simulink model "AeroCoeffsNew"  (R2020b)
settings: Solver=VariableStepAuto  StartTime=0.0  StopTime=50  FixedStep=0.1  RelTol=1e-3
values from neighbouring files (symbols this model uses):
  A_2 = [0  0  0; 0  0  0; 0  0  0]    [Angular_gust.mat]    (also in Linear_gust.mat; Real_Values.m = zeros(3); Trial_Script.m = zeros(3); TryingNewAeroCoeffs.m = zeros(3))
  A_kal = [0 0 0 0 0 0 0 0 0 0 0 0 ... (36 elements, 6x6)]    [Angular_gust.mat]    (also in Linear_gust.mat; Real_Values.m = [0 0 0 1 0 0; Trial_Script.m = [0 0 0 1 0 0; TryingNewAeroCoeffs.m = [0 0 0 1 0 0)
  B_2 = [0.0024294842205  2.57653534931e-06  6.44659625064e-05; 0  -0.000916808772026  -2.10833406567e-07; 0  0  -0.000799328564006]    [Angular_gust.mat]    (also in Linear_gust.mat; Real_Values.m = I_inv; Trial_Script.m = I_inv; TryingNewAeroCoeffs.m = I_inv)
  B_kal = [0 0 0 0 0 0 0 0 0 0 0 0 ... (36 elements, 6x6)]    [Angular_gust.mat]    (also in Linear_gust.mat; Real_Values.m = [0 0 0 0 0 0; Trial_Script.m = [0 0 0 0 0 0; TryingNewAeroCoeffs.m = [0 0 0 0 0 0)
  C_2 = [1  0  0; 0  1  0; 0  0  1]    [Angular_gust.mat]    (also in Linear_gust.mat; Real_Values.m = eye(3); Trial_Script.m = eye(3); TryingNewAeroCoeffs.m = eye(3))
  C_kal = [1 0 0 0 0 0 0 1 0 0 0 0 ... (36 elements, 6x6)]    [Angular_gust.mat]    (also in Linear_gust.mat; Real_Values.m = eye(6); Trial_Script.m = eye(6); TryingNewAeroCoeffs.m = eye(6))
  D_2 = [0  0  0; 0  0  0; 0  0  0]    [Angular_gust.mat]    (also in Linear_gust.mat; Real_Values.m = zeros(3); Trial_Script.m = zeros(3); TryingNewAeroCoeffs.m = zeros(3))
  D_kal = [0 0 0 0 0 0 0 0 0 0 0 0 ... (36 elements, 6x6)]    [Angular_gust.mat]    (also in Linear_gust.mat; Real_Values.m = zeros(6); Trial_Script.m = zeros(6); TryingNewAeroCoeffs.m = zeros(6))
  delta_time = 0.0178961433409    [Angular_gust.mat]    (also in Linear_gust.mat; Real_Values.m = time/length(xdata); Trial_Script.m = time/length(xdata); TryingNewAeroCoeffs.m = time/length(xdata))
  Fb1_l = -2600    [Angular_gust.mat]    (also in Linear_gust.mat; Real_Values.m = -260; Trial_Script.m; TryingNewAeroCoeffs.m)
  Fb1_u = 2600    [Angular_gust.mat]    (also in Linear_gust.mat; Real_Values.m = 260; Trial_Script.m; TryingNewAeroCoeffs.m)
  Fb2_l = -2600    [Angular_gust.mat]    (also in Linear_gust.mat; Real_Values.m = -260; Trial_Script.m; TryingNewAeroCoeffs.m)
  Fb2_u = 2600    [Angular_gust.mat]    (also in Linear_gust.mat; Real_Values.m = 260; Trial_Script.m; TryingNewAeroCoeffs.m)
  Fb3_l = -3200    [Angular_gust.mat]    (also in Linear_gust.mat; Real_Values.m = -320; Trial_Script.m; TryingNewAeroCoeffs.m)
  Fb3_u = 3200    [Angular_gust.mat]    (also in Linear_gust.mat; Real_Values.m = 320; Trial_Script.m; TryingNewAeroCoeffs.m)
  Fb4_l = -3200    [Angular_gust.mat]    (also in Linear_gust.mat; Real_Values.m = -320; Trial_Script.m; TryingNewAeroCoeffs.m)
  Fb4_u = 3200    [Angular_gust.mat]    (also in Linear_gust.mat; Real_Values.m = 320; Trial_Script.m; TryingNewAeroCoeffs.m)
  Fc1_l = -300    [Angular_gust.mat]    (also in Linear_gust.mat; Real_Values.m = -100; Trial_Script.m = -3000; TryingNewAeroCoeffs.m)
  Fc1_u = 300    [Angular_gust.mat]    (also in Linear_gust.mat; Real_Values.m = 100; Trial_Script.m = 3000; TryingNewAeroCoeffs.m)
  Fc2_l = -300    [Angular_gust.mat]    (also in Linear_gust.mat; Real_Values.m = -100; Trial_Script.m = -3000; TryingNewAeroCoeffs.m)
  Fc2_u = 300    [Angular_gust.mat]    (also in Linear_gust.mat; Real_Values.m = 100; Trial_Script.m = 3000; TryingNewAeroCoeffs.m)
  Fc3_l = -300    [Angular_gust.mat]    (also in Linear_gust.mat; Real_Values.m = -100; Trial_Script.m = -3000; TryingNewAeroCoeffs.m)
  Fc3_u = 300    [Angular_gust.mat]    (also in Linear_gust.mat; Real_Values.m = 100; Trial_Script.m = 3000; TryingNewAeroCoeffs.m)
  fprop = 1000    [Angular_gust.mat]    (also in Linear_gust.mat; TryingNewAeroCoeffs.m)
  Ft1_l = -5600    [Angular_gust.mat]    (also in Linear_gust.mat; Real_Values.m = -560; Trial_Script.m; TryingNewAeroCoeffs.m)
  Ft1_u = 5600    [Angular_gust.mat]    (also in Linear_gust.mat; Real_Values.m = 560; Trial_Script.m; TryingNewAeroCoeffs.m)
  Ft2_l = -5600    [Angular_gust.mat]    (also in Linear_gust.mat; Real_Values.m = -560; Trial_Script.m; TryingNewAeroCoeffs.m)
  Ft2_u = 5600    [Angular_gust.mat]    (also in Linear_gust.mat; Real_Values.m = 560; Trial_Script.m; TryingNewAeroCoeffs.m)
  Ft3_l = -3200    [Angular_gust.mat]    (also in Linear_gust.mat; Real_Values.m = -320; Trial_Script.m; TryingNewAeroCoeffs.m)
  Ft3_u = 3200    [Angular_gust.mat]    (also in Linear_gust.mat; Real_Values.m = 320; Trial_Script.m; TryingNewAeroCoeffs.m)
  Ft4_l = -3200    [Angular_gust.mat]    (also in Linear_gust.mat; Real_Values.m = -320; Trial_Script.m; TryingNewAeroCoeffs.m)
  Ft4_u = 3200    [Angular_gust.mat]    (also in Linear_gust.mat; Real_Values.m = 320; Trial_Script.m; TryingNewAeroCoeffs.m)
  g = 9.81    [Angular_gust.mat]    (also in Linear_gust.mat; Real_Values.m; Trial_Script.m; TryingNewAeroCoeffs.m)
  m = 941.102    [Angular_gust.mat]    (also in Linear_gust.mat; Real_Values.m; Trial_Script.m = 645; TryingNewAeroCoeffs.m)
  r_0 = [0 0 0]    [Angular_gust.mat]    (also in Linear_gust.mat; Real_Values.m = [0;0;0]; Trial_Script.m = [0;0;0]; TryingNewAeroCoeffs.m = [0;0;0])
  r_cgCatia = [0.0401998 0.00180957 -0.293434]    [Angular_gust.mat]    (also in Linear_gust.mat; Real_Values.m = TcgCatia*r_cgCatia; Trial_Script.m = [2; 0; 0]; TryingNewAeroCoeffs.m = TcgCatia*r_cgCatia)
  r_trajectory = [0 0 0]    [Angular_gust.mat]    (also in Linear_gust.mat; Real_Values.m = [0;0;0]; Trial_Script.m = [0;0;0]; TryingNewAeroCoeffs.m = [0;0;0])
  rho = 1.225    [Angular_gust.mat]    (also in Linear_gust.mat; Real_Values.m; Trial_Script.m; TryingNewAeroCoeffs.m)
  T = 10.5    [Angular_gust.mat]    (also in Linear_gust.mat; Real_Values.m; Trial_Script.m; TryingNewAeroCoeffs.m)
  t_finalgust = 17.9140394843    [Angular_gust.mat]    (also in Linear_gust.mat; Real_Values.m = time; TryingNewAeroCoeffs.m = time)
  TcgCatia = [1  0  0; 0  -1  0; 0  0  -1]    [Angular_gust.mat]    (also in Linear_gust.mat; Real_Values.m = [1 0 0; Trial_Script.m = [1 0 0; TryingNewAeroCoeffs.m = [1 0 0)
  time = 17.9140394843    [Angular_gust.mat]    (also in Linear_gust.mat; Real_Values.m = rdiff_abs/V0_shard; Trial_Script.m = abs(rdiff_shard(2)/V0_shard(2)); TryingNewAeroCoeffs.m = rdiff_abs/V0_shard)
  time_delay = 0.01    [Angular_gust.mat]    (also in Linear_gust.mat; Real_Values.m = 0.1; Trial_Script.m = 0.1; TryingNewAeroCoeffs.m)
  Tzy_Shard = [6.12323399574e-17  1  1.22464679915e-16; 1  -6.12323399574e-17  -7.49879891331e-33; 0  1.22464679915e-16  -1]    [Angular_gust.mat]    (also in Linear_gust.mat; Real_Values.m = [cos(pi/2) -sin(pi/2) 0; sin(pi/2) cos(pi/2) 0; 0 0 1]*[1 0 ; Trial_Script.m = [cos(pi/2) -sin(pi/2) 0; sin(pi/2) cos(pi/2) 0; 0 0 1]*[1 0 ; TryingNewAeroCoeffs.m = [cos(pi/2) -sin(pi/2) 0; sin(pi/2) cos(pi/2) 0; 0 0 1]*[1 0 )
  u0_final = 23.9559    [Angular_gust.mat]    (also in Linear_gust.mat; Real_Values.m = u_0(length(u_0)); TryingNewAeroCoeffs.m = u_0(length(u_0)))
  u1_final = -0.480858    [Angular_gust.mat]    (also in Linear_gust.mat; Real_Values.m = u_1(length(u_1)); TryingNewAeroCoeffs.m = u_1(length(u_1)))
  u2_final = -0.725589    [Angular_gust.mat]    (also in Linear_gust.mat; Real_Values.m = u_2(length(u_2)); TryingNewAeroCoeffs.m = u_2(length(u_2)))
  u_0 = [24.7775 24.7775 24.7775 24.7775 24.7775 24.7775 24.7775 24.7775 24.7775 24.7775 24.7775 24.7775 ... (1001 elements, 1001x1)]    [Angular_gust.mat]    (also in Linear_gust.mat; Real_Values.m = a(1:d_shard,1); Trial_Script.m = a(1:d_shard,1); TryingNewAeroCoeffs.m = a(1:d_shard,1))
  u_1 = [0.712897 0.712897 0.712897 0.712897 0.712897 0.712897 0.712897 0.712897 0.712897 0.712897 0.712897 0.712897 ... (1001 elements, 1001x1)]    [Angular_gust.mat]    (also in Linear_gust.mat; Real_Values.m = a(1:d_shard,2); Trial_Script.m = a(1:d_shard,2); TryingNewAeroCoeffs.m = a(1:d_shard,2))
  u_2 = [-0.504815 -0.504815 -0.504815 -0.504815 -0.504815 -0.504815 -0.504815 -0.504815 -0.504815 -0.504815 -0.504815 -0.504815 ... (1001 elements, 1001x1)]    [Angular_gust.mat]    (also in Linear_gust.mat; Real_Values.m = a(1:d_shard,3); Trial_Script.m = a(1:d_shard,3); TryingNewAeroCoeffs.m = a(1:d_shard,3))
  v_0 = [0 0 0]    [Angular_gust.mat]    (also in Linear_gust.mat; Real_Values.m = [0;0;0]; Trial_Script.m = [0;0;0]; TryingNewAeroCoeffs.m = [0;0;0])
  ZI_Cx = [4.10002314469 4.10486511138 4.10970707807 4.11454904475 4.11939101144 4.12423297813 4.12907494481 4.1339169115 4.13875887819 4.14360084487 4.14844281156 4.15328477825 ... (65341 elements, 361x181)]    [Angular_gust.mat]    (also in Linear_gust.mat; Real_Values.m = model_Cx(XI_Cx, YI_Cx); Trial_Script.m = model_Cx(XI_Cx, YI_Cx); TryingNewAeroCoeffs.m = model_Cx(XI_Cx, YI_Cx))
  ZI_Cy = [5.10662222372 5.15407485934 5.20152749496 5.24898013059 5.29643276621 5.34388540184 5.39133803746 5.43879067308 5.48624330871 5.53369594433 5.58114857996 5.62860121558 ... (65341 elements, 361x181)]    [Angular_gust.mat]    (also in Linear_gust.mat; Real_Values.m = model_Cy(XI_Cy, YI_Cy); Trial_Script.m = model_Cy(XI_Cy, YI_Cy); TryingNewAeroCoeffs.m = model_Cy(XI_Cy, YI_Cy))
  ZI_Cz = [-10.5947720774 -10.6317912004 -10.6688103235 -10.7058294465 -10.7428485695 -10.7798676926 -10.8168868156 -10.8539059387 -10.8909250617 -10.9279441847 -10.9649633078 -11.0019824308 ... (65341 elements, 361x181)]    [Angular_gust.mat]    (also in Linear_gust.mat; Real_Values.m = model_Cz(XI_Cz, YI_Cz); Trial_Script.m = model_Cz(XI_Cz, YI_Cz); TryingNewAeroCoeffs.m = model_Cz(XI_Cz, YI_Cz))
  ZI_p = [6.05111971338 6.06712776392 6.08313581446 6.099143865 6.11515191553 6.13115996607 6.14716801661 6.16317606715 6.17918411769 6.19519216823 6.21120021877 6.22720826931 ... (65341 elements, 361x181)]    [Angular_gust.mat]    (also in Linear_gust.mat; Real_Values.m = model_p(XI_p, YI_p); Trial_Script.m = model_p(XI_p, YI_p); TryingNewAeroCoeffs.m = model_p(XI_p, YI_p))
  ZI_q = [0.071083987219 0.054175962948 0.0372679386771 0.0203599144061 0.00345189013513 -0.0134561341358 -0.0303641584068 -0.0472721826778 -0.0641802069487 -0.0810882312197 -0.0979962554907 -0.114904279762 ... (65341 elements, 361x181)]    [Angular_gust.mat]    (also in Linear_gust.mat; Real_Values.m = model_q(XI_q, YI_q); Trial_Script.m = model_q(XI_q, YI_q); TryingNewAeroCoeffs.m = model_q(XI_q, YI_q))
  ZI_r = [-1.8762921931 -1.88364224017 -1.89099228723 -1.8983423343 -1.90569238136 -1.91304242842 -1.92039247549 -1.92774252255 -1.93509256961 -1.94244261668 -1.94979266374 -1.95714271081 ... (65341 elements, 361x181)]    [Angular_gust.mat]    (also in Linear_gust.mat; Real_Values.m = model_r(XI_r, YI_r); Trial_Script.m = model_r(XI_r, YI_r); TryingNewAeroCoeffs.m = model_r(XI_r, YI_r))
undefined symbols (not defined in the file or in its folder): Continuous, Time
libraries: dspsigops x11, simulink x9, fuzblock x3, pid_lib x3, sharedutil x1, mpclib x1, cstblocks x1, dspmathops x1, ctrlSharedLib x1
(part 2 of 2)

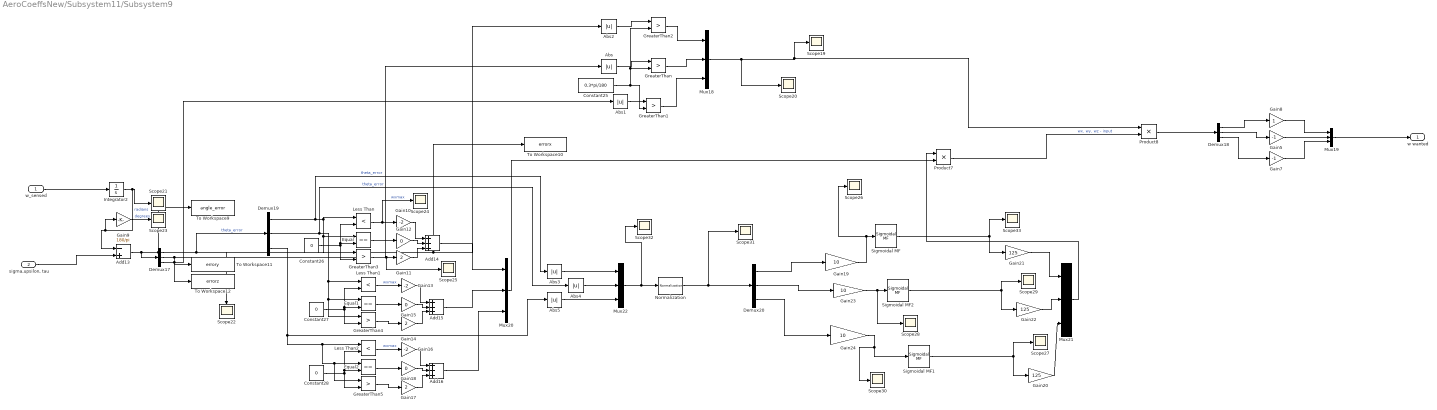
== system AeroCoeffsNew/Subsystem11/Subsystem9 ==
  w_sensed : Inport
  "sigma,upsilon, tau" : Inport  Port=2
  Abs{,1..5} (6 alike) : Abs
  Add13 : Sum  Inputs=-+
  Add14 : Sum  Inputs=+++
  Add15 : Sum  Inputs=+++
  Add16 : Sum  Inputs=+++
  Constant25 : Constant  Value=0.3*pi/180
  Constant26 : Constant  Value=0
  Constant27 : Constant  Value=0
  Constant28 : Constant  Value=0
  Demux{17..20} (4 alike) : Demux  Outputs=3
  Equal : RelationalOperator  Operator===  OutDataTypeStr=boolean  RndMeth=Simplest
  Equal1 : RelationalOperator  Operator===  OutDataTypeStr=boolean  RndMeth=Simplest
  Equal2 : RelationalOperator  Operator===  OutDataTypeStr=boolean  RndMeth=Simplest
  Gain10 : Gain  Gain=-2
  Gain11 : Gain  Gain=2
  Gain12 : Gain  Gain=0
  Gain13 : Gain  Gain=-2
  Gain14 : Gain  Gain=2
  Gain15 : Gain  Gain=0
  Gain16 : Gain  Gain=-2
  Gain17 : Gain  Gain=2
  Gain18 : Gain  Gain=0
  Gain19 : Gain  Gain=10
  Gain20 : Gain  Gain=125
  Gain21 : Gain  Gain=125
  Gain22 : Gain  Gain=125
  Gain23 : Gain  Gain=10
  Gain24 : Gain  Gain=10
  Gain5 : Gain  Gain=-1
  Gain7 : Gain  Gain=-1
  Gain8 : Gain
  Gain9 : Gain  Gain=180/pi
  GreaterThan{,1..5} (6 alike) : RelationalOperator  Operator=>  OutDataTypeStr=boolean  RndMeth=Simplest
  Integrator2 : Integrator  InitialCondition=[0;0;0]
  Less Than : RelationalOperator  Operator=<  OutDataTypeStr=boolean  RndMeth=Simplest
  Less Than1 : RelationalOperator  Operator=<  OutDataTypeStr=boolean  RndMeth=Simplest
  Less Than2 : RelationalOperator  Operator=<  OutDataTypeStr=boolean  RndMeth=Simplest
  Mux{18..22} (5 alike) : Mux  Inputs=3
  Normalization : dspmathops/Normalization  NormType=Squared 2-norm  Bias=1e-10  NormOver=Each column  Dimension=1  roundingMode=Floor  overflowMode=off  accumDataTypeStr=Inherit: Same as product output  accumLastDataTypeStr=Inherit: Same as product output  outputDataTypeStr=Inherit: Same as product output  outputMin=[]  outputMax=[]  outputLastDataTypeStr=Inherit: Same as product output
  Product7 : Product
  Product8 : Product
  Scope{19..33} (15 alike) : Scope
  Sigmoidal MF : fuzblock/Membership  Functions/Sigmoidal MF  a=10^(-8)  c=1000
      settings: SourceProductBaseCode=FL
  Sigmoidal MF1 : fuzblock/Membership  Functions/Sigmoidal MF  a=10^(-8)  c=1000
      settings: SourceProductBaseCode=FL
  Sigmoidal MF2 : fuzblock/Membership  Functions/Sigmoidal MF  a=10^(-8)  c=1000
      settings: SourceProductBaseCode=FL
  To Workspace10 : ToWorkspace  VariableName=errorx  SaveFormat=Timeseries  SampleTime=-1
      settings: Save2DSignal=2-D array (concatenate along first dimension)
  To Workspace11 : ToWorkspace  VariableName=errory  SaveFormat=Timeseries  SampleTime=-1
  To Workspace12 : ToWorkspace  VariableName=errorz  SaveFormat=Timeseries  SampleTime=-1
  To Workspace9 : ToWorkspace  VariableName=angle_error  SampleTime=-1
  w wanted : Outport
  wires:
  Normalization/1 -> Scope31/1, Demux20/1
  Demux19/2 -> Abs4/1, GreaterThan4/1, Equal1/1, Less Than1/1  "theta_error"
  Less Than1/1 -> Gain13/1  "wxmax"
  Gain9/1 -> Scope23/1  "degrees"
  Gain7/1 -> Mux19/3
  Constant28/1 -> Equal2/2, Less Than2/2, GreaterThan5/2
  Gain16/1 -> Add16/1
  Sigmoidal MF1/1 -> Gain20/1, Scope27/1
  Constant27/1 -> Equal1/2, Less Than1/2, GreaterThan4/2
  Demux17/2 -> Abs/1, To Workspace11/1
  Demux18/2 -> Gain5/1
  Mux21/1 -> Product7/1
  Demux18/1 -> Gain8/1
  Constant26/1 -> Equal/2, Less Than/2, GreaterThan3/2
  w_sensed/1 -> Integrator2/1
  Gain20/1 -> Mux21/3
  GreaterThan/1 -> Mux18/2
  Gain11/1 -> Add14/3
  Equal/1 -> Gain12/1
  Abs2/1 -> GreaterThan2/1
  Demux19/3 -> Abs5/1, GreaterThan5/1, Equal2/1, Less Than2/1
  GreaterThan5/1 -> Gain17/1
  Demux19/1 -> Abs3/1, GreaterThan3/1, Equal/1, Less Than/1  "theta_error"
  Gain23/1 -> Scope28/1, Sigmoidal MF2/1
  Constant25/1 -> GreaterThan2/2, GreaterThan/2, GreaterThan1/2
  Mux18/1 -> Product8/1, Scope19/1, Scope20/1
  Mux22/1 -> Scope32/1, Normalization/1
  Add15/1 -> Mux20/2
  Integrator2/1 -> Add13/1, Gain9/1, Scope21/1  "radians"
  Product8/1 -> Demux18/1
  Add13/1 -> Demux19/1, Scope22/1, To Workspace9/1, Demux17/1  "theta_error"
  Gain8/1 -> Mux19/1
  Gain5/1 -> Mux19/2
  GreaterThan1/1 -> Mux18/3
  GreaterThan2/1 -> Mux18/1
  Mux20/1 -> Product7/2
  Less Than/1 -> Scope24/1, Gain10/1  "wxmax"
  Equal2/1 -> Gain18/1
  Add16/1 -> Mux20/3
  Gain13/1 -> Add15/1
  Demux20/1 -> Gain19/1
  Less Than2/1 -> Gain16/1  "wxmax"
  Gain17/1 -> Add16/3
  Product7/1 -> Product8/2  "wx, wy, wz - input"
  Gain10/1 -> Add14/1
  Gain12/1 -> Add14/2
  Equal1/1 -> Gain15/1
  Gain18/1 -> Add16/2
  Gain21/1 -> Mux21/1
  Demux17/3 -> Abs1/1, To Workspace12/1
  GreaterThan4/1 -> Gain14/1
  Gain15/1 -> Add15/2
  Add14/1 -> Mux20/1
  Demux17/1 -> Abs2/1, To Workspace10/1
  Gain22/1 -> Mux21/2
  GreaterThan3/1 -> Scope25/1, Gain11/1
  Demux18/3 -> Gain7/1
  Gain14/1 -> Add15/3
  Demux20/3 -> Gain24/1
  Abs1/1 -> GreaterThan1/1
  Abs5/1 -> Mux22/3
  Sigmoidal MF/1 -> Gain21/1, Scope33/1
  Abs3/1 -> Mux22/1
  Sigmoidal MF2/1 -> Gain22/1, Scope29/1
  Gain19/1 -> Scope26/1, Sigmoidal MF/1
  Abs/1 -> GreaterThan/1
  Gain24/1 -> Scope30/1, Sigmoidal MF1/1
  Abs4/1 -> Mux22/2
  Demux20/2 -> Gain23/1
  Mux19/1 -> w wanted/1
  "sigma,upsilon, tau"/1 -> Add13/2

== system AeroCoeffsNew/Subsystem5/Subsystem ==
  F_c_d : Inport
  M_c_d : Inport  Port=2
  Demux8 : Demux  Outputs=3
  Demux9 : Demux  Outputs=3
  MATLAB Function : MATLAB Function  TreatAsAtomicUnit=on
  MATLAB Function6 : MATLAB Function  TreatAsAtomicUnit=on
  Mux23 : Mux
  Mux24 : Mux
  Mux9 : Mux  Inputs=3
  Terminator12 : Terminator
  To Workspace6 : ToWorkspace  VariableName=Fc_wanted  SaveFormat=Timeseries  SampleTime=-1
  To Workspace7 : ToWorkspace  VariableName=Ft_wanted  SaveFormat=Timeseries  SampleTime=-1
  To Workspace8 : ToWorkspace  VariableName=Fb_wanted  SaveFormat=Timeseries  SampleTime=-1
  Fb_wanted : Outport
  Ft_wanted : Outport  Port=2
  Fc_wanted : Outport  Port=3
  wires:
  Demux9/3 -> MATLAB Function6/3(M_z)
  Demux8/2 -> MATLAB Function6/1(F_y)
  Mux9/1 -> Fc_wanted/1, To Workspace6/1  "Fc_wanted"
  MATLAB Function/2(Ft2) -> Mux23/2  "Fb_wanted"
  Demux9/1 -> MATLAB Function6/2(M_x)
  MATLAB Function/3(Ft3) -> Mux23/3
  Demux9/2 -> MATLAB Function/1(My)
  MATLAB Function/8(Fb4) -> Mux24/4
  MATLAB Function6/1(F_c1) -> Mux9/1
  MATLAB Function/1(Ft1) -> Mux23/1  "Ft_wanted"
  Demux8/1 -> Terminator12/1
  Mux23/1 -> Ft_wanted/1, To Workspace7/1  "Ft_wanted"
  Mux24/1 -> Fb_wanted/1, To Workspace8/1  "Fb_wanted"
  MATLAB Function6/3(F_c3) -> Mux9/3
  MATLAB Function/5(Fb1) -> Mux24/1
  MATLAB Function/6(Fb2) -> Mux24/2
  MATLAB Function/7(Fb3) -> Mux24/3
  MATLAB Function/4(Ft4) -> Mux23/4
  Demux8/3 -> MATLAB Function/2(Fz)
  MATLAB Function6/2(F_c2) -> Mux9/2
  F_c_d/1 -> Demux8/1
  M_c_d/1 -> Demux9/1

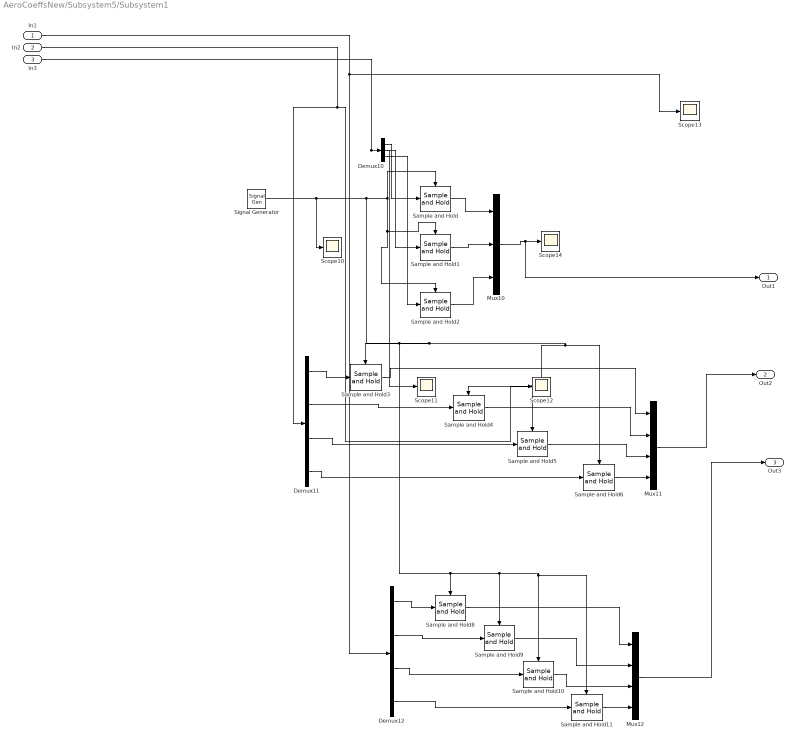
== system AeroCoeffsNew/Subsystem5/Subsystem1 ==
  In1 : Inport
  In2 : Inport  Port=2
  In3 : Inport  Port=3
  Demux10 : Demux  Outputs=3
  Demux11 : Demux
  Demux12 : Demux
  Mux10 : Mux  Inputs=3
  Mux11 : Mux
  Mux12 : Mux
  Sample and Hold{,1..6,8..11} (11 alike) : dspsigops/Sample and Hold  trig=Rising edge  initCond=0  latchinput=off
  Scope{10..14} (5 alike) : Scope
  Signal Generator : SignalGenerator  WaveForm=square  Frequency=fprop  Units=rad/sec
  Out1 : Outport
  Out2 : Outport  Port=2
  Out3 : Outport  Port=3
  wires:
  Demux12/1 -> Sample and Hold8/1
  Demux11/1 -> Sample and Hold3/1
  Signal Generator/1 -> Scope10/1, Sample and Hold11/Trigger, Sample and Hold10/Trigger, Sample and Hold9/Trigger, Sample and Hold8/Trigger, Sample and Hold4/Trigger, Sample and Hold5/Trigger, Sample and Hold6/Trigger, Sample and Hold3/Trigger, Sample and Hold/Trigger, Sample and Hold2/Trigger, Sample and Hold1/Trigger
  In2/1 -> Scope12/1, Demux11/1
  In3/1 -> Scope11/1, Demux10/1
  Demux10/3 -> Sample and Hold2/1
  Sample and Hold10/1 -> Mux12/3
  Sample and Hold/1 -> Mux10/1
  Demux12/4 -> Sample and Hold11/1
  Sample and Hold6/1 -> Mux11/4
  Demux10/1 -> Sample and Hold/1
  Mux10/1 -> Out1/1, Scope14/1
  Demux12/3 -> Sample and Hold10/1
  Sample and Hold8/1 -> Mux12/1
  Sample and Hold3/1 -> Mux11/1
  Sample and Hold5/1 -> Mux11/3
  Sample and Hold1/1 -> Mux10/2
  Sample and Hold11/1 -> Mux12/4
  In1/1 -> Scope13/1, Demux12/1
  Demux10/2 -> Sample and Hold1/1
  Demux11/2 -> Sample and Hold4/1
  Sample and Hold2/1 -> Mux10/3
  Sample and Hold4/1 -> Mux11/2
  Sample and Hold9/1 -> Mux12/2
  Demux11/3 -> Sample and Hold5/1
  Mux12/1 -> Out3/1
  Demux12/2 -> Sample and Hold9/1
  Demux11/4 -> Sample and Hold6/1
  Mux11/1 -> Out2/1

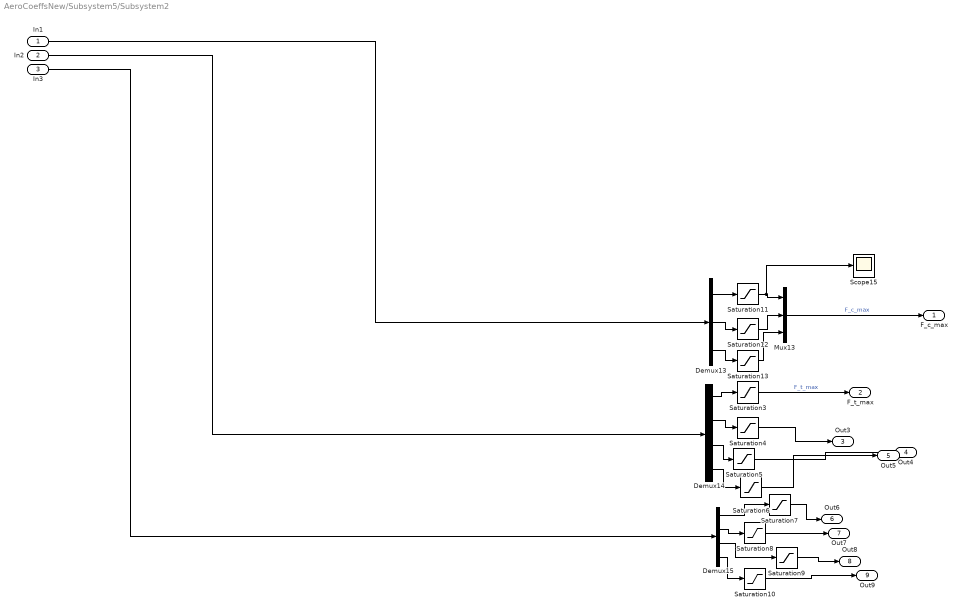
== system AeroCoeffsNew/Subsystem5/Subsystem2 ==
  In1 : Inport
  In2 : Inport  Port=2
  In3 : Inport  Port=3
  Demux13 : Demux  Outputs=3
  Demux14 : Demux
  Demux15 : Demux
  Mux13 : Mux  Inputs=3
  Saturation10 : Saturate  UpperLimit=Fb4_u  LowerLimit=Fb4_l
  Saturation11 : Saturate  UpperLimit=Fc1_u  LowerLimit=Fc1_l
  Saturation12 : Saturate  UpperLimit=Fc2_u  LowerLimit=Fc2_l
  Saturation13 : Saturate  UpperLimit=Fc3_u  LowerLimit=Fc3_l
  Saturation3 : Saturate  UpperLimit=Ft1_u  LowerLimit=Ft1_l
  Saturation4 : Saturate  UpperLimit=Ft2_u  LowerLimit=Ft2_l
  Saturation5 : Saturate  UpperLimit=Ft3_u  LowerLimit=Ft3_l
  Saturation6 : Saturate  UpperLimit=Ft4_u  LowerLimit=Ft4_l
  Saturation7 : Saturate  UpperLimit=Fb1_u  LowerLimit=Fb1_l
  Saturation8 : Saturate  UpperLimit=Fb2_u  LowerLimit=Fb2_l
  Saturation9 : Saturate  UpperLimit=Fb3_u  LowerLimit=Fb3_l
  Scope15 : Scope
  F_c_max : Outport
  F_t_max : Outport  Port=2
  Out3 : Outport  Port=3
  Out4 : Outport  Port=4
  Out5 : Outport  Port=5
  Out6 : Outport  Port=6
  Out7 : Outport  Port=7
  Out8 : Outport  Port=8
  Out9 : Outport  Port=9
  wires:
  Saturation11/1 -> Scope15/1, Mux13/1
  Demux13/2 -> Saturation12/1
  Saturation10/1 -> Out9/1
  Demux13/3 -> Saturation13/1
  Demux14/1 -> Saturation3/1
  Demux14/4 -> Saturation6/1
  In3/1 -> Demux15/1
  Demux14/3 -> Saturation5/1
  Demux13/1 -> Saturation11/1
  Saturation13/1 -> Mux13/3
  In1/1 -> Demux13/1
  Demux15/1 -> Saturation7/1
  Demux15/2 -> Saturation8/1
  Demux15/3 -> Saturation9/1
  Saturation12/1 -> Mux13/2
  Demux15/4 -> Saturation10/1
  Demux14/2 -> Saturation4/1
  Saturation9/1 -> Out8/1
  Saturation5/1 -> Out4/1
  In2/1 -> Demux14/1
  Saturation4/1 -> Out3/1
  Saturation7/1 -> Out6/1
  Mux13/1 -> F_c_max/1  "F_c_max"
  Saturation6/1 -> Out5/1
  Saturation3/1 -> F_t_max/1  "F_t_max"
  Saturation8/1 -> Out7/1

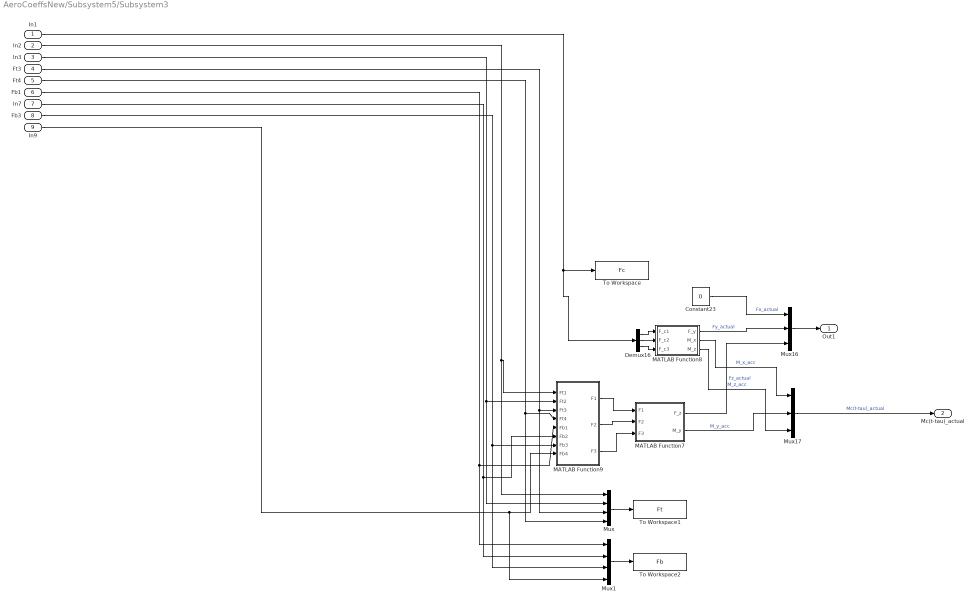
== system AeroCoeffsNew/Subsystem5/Subsystem3 ==
  In1 : Inport
  In2 : Inport  Port=2
  In3 : Inport  Port=3
  Ft3 : Inport  Port=4
  Ft4 : Inport  Port=5
  Fb1 : Inport  Port=6
  In7 : Inport  Port=7
  Fb3 : Inport  Port=8
  In9 : Inport  Port=9
  Constant23 : Constant  Value=0
  Demux16 : Demux  Outputs=3
  MATLAB Function7 : MATLAB Function  TreatAsAtomicUnit=on
  MATLAB Function8 : MATLAB Function  TreatAsAtomicUnit=on
  MATLAB Function9 : MATLAB Function  TreatAsAtomicUnit=on
  Mux : Mux
  Mux1 : Mux
  Mux16 : Mux  Inputs=3
  Mux17 : Mux  Inputs=3
  To Workspace : ToWorkspace  VariableName=Fc  SaveFormat=Timeseries  SampleTime=-1
  To Workspace1 : ToWorkspace  VariableName=Ft  SaveFormat=Timeseries  SampleTime=-1
  To Workspace2 : ToWorkspace  VariableName=Fb  SaveFormat=Timeseries  SampleTime=-1
  Out1 : Outport
  Mc(t-tau)_actual : Outport  Port=2
  wires:
  Demux16/2 -> MATLAB Function8/2(F_c2)
  In9/1 -> Mux1/4, MATLAB Function9/8(Fb4)
  In3/1 -> Mux/2, MATLAB Function9/2(Ft2)
  MATLAB Function7/1(F_z) -> Mux16/3  "Fz_actual"
  In1/1 -> Demux16/1, To Workspace/1
  Fb3/1 -> Mux1/3, MATLAB Function9/7(Fb3)
  MATLAB Function9/1(F1) -> MATLAB Function7/1(F1)
  Ft3/1 -> Mux/3, MATLAB Function9/3(Ft3)
  MATLAB Function8/1(F_y) -> Mux16/2  "Fy_actual"
  Fb1/1 -> Mux1/1, MATLAB Function9/5(Fb1)
  MATLAB Function8/3(M_z) -> Mux17/3  "M_z_acc"
  MATLAB Function7/2(M_y) -> Mux17/2  "M_y_acc"
  Mux17/1 -> Mc(t-tau)_actual/1  "Mc(t-tau)_actual"
  Ft4/1 -> Mux/4, MATLAB Function9/4(Ft4)
  MATLAB Function8/2(M_x) -> Mux17/1  "M_x_acc"
  In7/1 -> Mux1/2, MATLAB Function9/6(Fb2)
  MATLAB Function9/3(F3) -> MATLAB Function7/3(F3)
  Demux16/1 -> MATLAB Function8/1(F_c1)
  Constant23/1 -> Mux16/1  "Fx_actual"
  In2/1 -> Mux/1, MATLAB Function9/1(Ft1)
  MATLAB Function9/2(F2) -> MATLAB Function7/2(F2)
  Mux1/1 -> To Workspace2/1
  Demux16/3 -> MATLAB Function8/3(F_c3)
  Mux/1 -> To Workspace1/1
  Mux16/1 -> Out1/1

== system AeroCoeffsNew/Subsystem5/Subsystem4 ==
  TVd : Inport
  In2 : Inport  Port=2
  Constant24 : Constant  Value=[0;1;1]
  Matrix Multiply3 : Product  Multiplication=Matrix(*)
  Product5 : Product
  Fc(t-tau)_actual : Outport
  Fc(t-tau)_actual1 : Outport  Port=2
  wires:
  Matrix Multiply3/1 -> Fc(t-tau)_actual1/1, Product5/2  "Fc(t-tau)_actual"
  Constant24/1 -> Product5/1
  TVd/1 -> Matrix Multiply3/1
  Product5/1 -> Fc(t-tau)_actual/1  "Fc(t-tau)_actual"
  In2/1 -> Matrix Multiply3/2

== system AeroCoeffsNew/Subsystem9/Subsystem6 ==
  Fc(t-tau) : Inport
  a_sensed : Inport  Port=2
  gps error : Inport  Port=3
  Constant8 : Constant  Value=0
  Demux2 : Demux  Outputs=6
  Integrator1 : Integrator  InitialCondition=v_0
  Kalman Filter : ctrlSharedLib/Kalman Filter  TimeDomain=Continuous-Time  UseCurrentEstimator=on  ModelSource=Individual A, B, C, D matrices  ModelSourceVariable=ss(0.95,1,1,0,1)  A=A_kal  B=B_kal  C=C_kal  D=D_kal  NumberOfStates=1  NumberOfInputs=1  NumberOfOutputs=1  InitialEstimateSource=Dialog  X0=[0;0;0;0;0;0]  P0=10  UseK=off  UseGH=off  NumberOfProcessNoiseInputs=1  G=1  TimeInvariantG=on  H=0  TimeInvariantH=on  Q=0.05  TimeInvariantQ=on  R=1  TimeInvariantR=on  N=0  TimeInvariantN=on  AddInputPort=on  AddEnablePort=off  OutputEstimatedY=off  OutputP=off  Ts=-1
  Mux1 : Mux
  Mux3 : Mux  Inputs=3
  Mux4 : Mux  Inputs=2
  Terminator : Terminator
  Terminator2 : Terminator
  Terminator3 : Terminator
  Transpose : Math  Operator=transpose  SaturateOnIntegerOverflow=on
  r_kalman : Outport
  wires:
  Integrator1/1 -> Mux4/2  "v_sensed"
  Demux2/2 -> Mux3/2
  Kalman Filter/1 -> Demux2/1
  Constant8/1 -> Mux1/1, Mux1/3, Mux1/2
  Transpose/1 -> Mux4/1  "r_sensed"
  Mux1/1 -> Kalman Filter/1
  Demux2/4 -> Terminator/1
  Demux2/1 -> Mux3/1
  Demux2/3 -> Mux3/3
  Mux4/1 -> Kalman Filter/2
  Demux2/5 -> Terminator3/1
  Demux2/6 -> Terminator2/1
  Fc(t-tau)/1 -> Mux1/4
  Mux3/1 -> r_kalman/1  "r_kalman"
  gps error/1 -> Transpose/1
  a_sensed/1 -> Integrator1/1

== matlab function AeroCoeffsNew/Subsystem5/Subsystem/MATLAB Function6 ==
  data: F_y input; F_c1 output; M_x input; M_z input; F_c2 output; F_c3 output
function [F_c1, F_c2, F_c3] = fcn(F_y, M_x, M_z)
%CATIA trans
TcgCatia = [1 0 0;
    0 -1 0;
    0 0 -1];

%Propeller arms - changed due to CATIA errors
c_1 = [-640.1998; 0; 506.566]*10^(-3);      %Control Back Top
c_2 = [-1040.1998; 0; -493.434]*10^(-3);    %Control Back Bottom
c_3 = [2259.8002; 0; -293.434]*10^(-3);     %Control Front

%Propeller arms - rotated
c_1 = TcgCatia*c_1;
c1 = transpose(c_1);
c_2 = TcgCatia*c_2;
c2 = transpose(c_2);
c_3 = TcgCatia*c_3;
c3 = transpose(c_3);

xc_1 = c1(1);
zc_1 = c1(3);

xc_2 = c2(1);
zc_2 = c2(3);

xc_3 = c3(1);
zc_3 = c3(3);

A_control = [1 1 1;
    zc_1 zc_2 zc_3;
    xc_1 xc_2 xc_3];
A_cinv = inv(A_control);
force_control = [F_y; M_x; M_z];
controlvec = A_cinv*force_control;
F_c1 = controlvec(1);
F_c2 = controlvec(2);
F_c3 = controlvec(3);
end

== matlab function AeroCoeffsNew/Subsystem5/MATLAB Function4 ==
  data: F1 input; F_t1 output; F2 input; F3 input; F_t2 output; F_t3 output; F_t4 output; F_b1 output; F_b2 output; F_b3 output; F_b4 output
function [F_t1, F_t2, F_t3, F_t4, F_b1, F_b2, F_b3, F_b4] = fcn(F1, F2, F3)
%F3 is one prop
%F1 is two props
%F2 is two props
F_t1 = F1/2;
F_t2 = F_t1;
F_t3 = F3;
F_t4 = F_t3;
F_b3 = F_t3;
F_b4 = F_t3;
F_b1 = F2/2;
F_b2 = F_b1;

Ft = [F_t1, F_t2, F_t3, F_t4];
Fb = [F_b1, F_b2, F_b3, F_b4];
end

== matlab function AeroCoeffsNew/Subsystem5/Subsystem3/MATLAB Function7 ==
  data: F1 input; F_z output; F2 input; M_y output; F3 input
function [F_z, M_y] = fcn(F1, F2, F3)
xt_1 = 1.2598;
xb_1 = 2.2598;
xt_3 = -1.3402;
x_t1 = xt_1;
x_b1 = xb_1;
x_t3 = xt_3;

M_y = -100;
F_z = 0;

A_mat = [1 1;
    xt_1 xb_1];

A_inv = inv(A_mat);

force = [F1; F2];

back = A_mat*force;
backtrack = [4*F3; 4*F3*xt_3];
forceback = back+backtrack;
F_z = forceback(1);
M_y = forceback(2) + 0.15;
end

== matlab function AeroCoeffsNew/Subsystem5/Subsystem3/MATLAB Function8 ==
  data: F_c1 input; F_y output; M_x output; F_c2 input; F_c3 input; M_z output
function [F_y, M_x, M_z] = fcn(F_c1, F_c2, F_c3)

%CATIA trans
TcgCatia = [1 0 0;
    0 -1 0;
    0 0 -1];

%Propeller arms - changed due to CATIA errors
c_1 = [-640.1998; 0; 506.566]*10^(-3);      %Control Back Top
c_2 = [-1040.1998; 0; -493.434]*10^(-3);    %Control Back Bottom
c_3 = [2259.8002; 0; -293.434]*10^(-3);     %Control Front

%Propeller arms - rotated
c_1 = TcgCatia*c_1;
c1 = transpose(c_1);
c_2 = TcgCatia*c_2;
c2 = transpose(c_2);
c_3 = TcgCatia*c_3;
c3 = transpose(c_3);

xc_1 = c1(1);
zc_1 = c1(3);

xc_2 = c2(1);
zc_2 = c2(3);

xc_3 = c3(1);
zc_3 = c3(3);


Control_forces = [F_c1; F_c2; F_c3];

A_control = [1 1 1;
        zc_1 zc_2 zc_3;
        xc_1 xc_2 xc_3]; 
Control_vec_2 = A_control*Control_forces;
F_y = Control_vec_2(1);
M_x = Control_vec_2(2);
M_z = Control_vec_2(3);
end

== matlab function AeroCoeffsNew/Subsystem5/Subsystem3/MATLAB Function9 ==
  data: Ft1 input; F1 output; Ft2 input; F2 output; F3 output; Ft3 input; Ft4 input; Fb1 input; Fb2 input; Fb3 input; Fb4 input
function [F1, F2, F3] = fcn(Ft1, Ft2, Ft3, Ft4, Fb1, Fb2, Fb3, Fb4)
%F3 is one prop
%F1 is two props
%F2 is two props
F1 = 2*Ft1;
F2 = 2*Fb1;
F3 = Ft3;
end

== matlab function AeroCoeffsNew/Subsystem4/MATLAB Function2 ==
  data: theta_x input; Transformation_Mat output; theta_y input; theta_z input
function Transformation_Mat  = Euler(theta_x, theta_y, theta_z)

a = cos(theta_x)*cos(theta_z);
b = cos(theta_x)*sin(theta_z);
c = - sin(theta_x);
d = sin(theta_y)*sin(theta_x)*cos(theta_z) - cos(theta_y)*sin(theta_z);
e = sin(theta_y)*sin(theta_x)*sin(theta_z) + cos(theta_y)*cos(theta_z);
f = sin(theta_y)*cos(theta_x);
g = cos(theta_y)*sin(theta_x)*cos(theta_z) + sin(theta_y)*sin(theta_z);
h = cos(theta_y)*sin(theta_x)*sin(theta_z) - sin(theta_y)*cos(theta_z);
i = cos(theta_y)*cos(theta_x);

Transformation_Mat = [a b c;
    d e f;
    g h i];


end

== matlab function AeroCoeffsNew/Subsystem9/GPS Model ==
  settings: updateMethod=DISCRETE
  data: position input; newposition output
function newposition  = gps(position)

    % Input: position
    % Output: position with gps accuracies inclduded
    mu = 0; 
    sigma = 0.015;

    r1 = normrnd(mu, sigma);
    r2 = normrnd(mu, sigma);
    r3 = normrnd(mu, sigma);

    newposition = [0,0,0];

    newposition(1) = position(1) + r1;
    newposition(2) = position(2) + r2;
    newposition(3) = position(3) + r3;

end

== matlab function AeroCoeffsNew/Subsystem4/MATLAB Function3 ==
  data: theta_x input; Transformation_Mat output; theta_y input; theta_z input
function Transformation_Mat  = Euler(theta_x, theta_y, theta_z)

a = cos(theta_x)*cos(theta_z);
b = cos(theta_x)*sin(theta_z);
c = - sin(theta_x);
d = sin(theta_y)*sin(theta_x)*cos(theta_z) - cos(theta_y)*sin(theta_z);
e = sin(theta_y)*sin(theta_x)*sin(theta_z) + cos(theta_y)*cos(theta_z);
f = sin(theta_y)*cos(theta_x);
g = cos(theta_y)*sin(theta_x)*cos(theta_z) + sin(theta_y)*sin(theta_z);
h = cos(theta_y)*sin(theta_x)*sin(theta_z) - sin(theta_y)*cos(theta_z);
i = cos(theta_y)*cos(theta_x);

Transformation_Mat = [a b c;
    d e f;
    g h i];


end

== matlab function AeroCoeffsNew/Subsystem5/Subsystem/MATLAB Function ==
  data: My input; Ft1 output; Fz input; Ft2 output; Ft3 output; Ft4 output; Fb1 output; Fb2 output; Fb3 output; Fb4 output
function [Ft1, Ft2, Ft3, Ft4, Fb1, Fb2, Fb3, Fb4] = fixingpropulsionsmess(My, Fz)
xt_1 = 1.2598;
xb_1 = 2.2598;
xt_3 = -1.3402;
xb_3 = -1.3402;
x_t1 = xt_1;
x_b1 = xb_1;
x_t3 = xt_3;
x_b3 = xb_3;;

%alpha_1 = (-2*xt_1*(1/((xt_1/xb_1)-1))*(2 - (2*xb_3/xb_1)) - 4*xb_3)^2;
%alpha_2 = ((1/((xt_1/xb_1)-1))*(2-(2*xb_3/xb_1)))^2;
%alpha = alpha_1 + alpha_2;

%beta_1 = 2*My*((1/(2*xb_1))*(1 - (xt_1/xb_1)*(1/((xt_1/xb_1) -1))));
%beta_2 = 2*My*(1/((xt_1/xb_1) -1))*(1/(2*xb_1))*(1/((xt_1/xb_1) -1))*(2 - ((2*xb_3)/x_b1));
%beta_3 = 2*Fz*(1/(2*xb_1)*xt_1*(1/(xt_1/xb_1 -1)));
%beta_4 = 2*Fz*(-1/2*(1/(xt_1/xb_1 -1))*(1/(xt_1/xb_1 -1))*(2-2*xb_3/xb_1));
%beta = beta_1 + beta_2 + beta_3 + beta_4;

%a = beta/(2*alpha);
%y = 1/(2*xb_1)*(My - 2*xt_1*(1/(xt_1/xb_1 -1))*(-0.5*Fz + 2*(2 - 2*xb_3/xb_1)*a + 1/(2*xb_1)*My) - 4*xb_3*a);
%x = (1/(xt_1/xb_1 -1))*(-0.5*Fz + (2 - 2*xb_3/xb_1)*a + 1/(2*xb_1)*My);

a_num = 2/((2*xb_1 - 2*xt_1)^2) *(2*(4*xt_1 - 4*xb_3)*(My - Fz*0.5)) + 2*Fz + (4*My - Fz*(2 + 4*xt_1 - 4*xb_3))/(2*xb_1 - 2*xt_1);
a_den = -(2/((2*xb_1 - 2*xt_1)^2)*2*((4*xt_1 - 4*xb_3)^2) + 10 + (8*(4*xt_1 - 4*xb_3))/(-2*xt_1 + 2*xb_1));
a = a_num/a_den;

y = 1/(-2*xt_1 + 2*xb_1)*(a*(4*xt_1 - 4*xb_3) + My - 0.5*Fz);
x = -y - 2*a + Fz/2;
z = a;

Ft1 = x;
Ft2 = Ft1;
Ft3 = a;
Ft4 = Ft3;
Fb1 = y;
Fb2 = Fb1;
Fb3 = Ft3;
Fb4 = Ft3;
end

== matlab function AeroCoeffsNew/Subsystem2/MATLAB Function1 ==
  settings: updateMethod=DISCRETE
  data: angvel input; accelData output; acc input
function accelData = accelerometer(angvel, acc)

    %
    % Create gyroscope sensor object
    params = accelparams;
    
    % Parameters for simulated signal
    N = 1;       % Number of samples
    Fs = 100000;       % Sampling rate
    %Fc = 0.25;      % Sinusoidal frequency
    
    
    % Create arrays
    t = (0:(1/Fs):((N-1)/Fs)).';
    acc = acc;          %Input accelerations
    orient = quaternion.ones(N, 1);
    angvel = angvel;
    
    % Generate acceleration data
    imu = imuSensor('SampleRate', Fs, 'Accelerometer', params);
    imu.Accelerometer.MeasurementRange = 1000;   % Maximum acceleration accelerometer can measure
    imu.Accelerometer.Resolution = 1/Fs;           % Step size of digital measurements
    
    % Biases
    imu.Accelerometer.BiasInstability = 0.000000000001; 7.5 / 1000 * 9.81;
    imu.Accelerometer.NoiseDensity = 0.000000000001;%150 / 1000 / 1000 * 9.81 /10; 
    imu.Accelerometer.TemperatureBias = 50 / 1000 / 1000 * 9.81;
    
  
    
    accelData = imu(acc, angvel, orient);
    
    accelData(:,3) = accelData(:,3) - 9.81;

    accelData(:,1) = accelData(:,1) * -1;
    accelData(:,2) = accelData(:,2) * -1;
    accelData(:,3) = accelData(:,3) * -1;

end

== matlab function AeroCoeffsNew/Subsystem3/MATLAB Function10 ==
  settings: updateMethod=DISCRETE
  data: xvel input; yvel input; zvel input; wx output; accx input; accy input; accz input; wy output; wz output
function [wx, wy, wz]  = fungyroscope(xvel, yvel, zvel, accx, accy, accz)
   
    % Create gyroscope sensor object
    params = gyroparams;         
    
    % Parameters for simulated signal
    N = 1;       % Number of samples
    Fs = 100;       % Sampling rate
    Fc = 0.25;      % Sinusoidal frequency
    
    % Create arrays
    t = (0:(1/Fs):((N-1)/Fs)).';
    acc = [accx, accy, accz];          % Input accelerations
    angvel = [xvel,yvel,zvel];
    %angvel(:,1) = 8*sin(2*pi*Fc*t);
    
    % Generate gyroscopic data
    imu = imuSensor('SampleRate', Fs, 'Gyroscope', params);
    %imu.Gyroscope.MeasurementRange = 1000;   % Maximum angular velocity gyroscope can measure
    %imu.Gyroscope.Resolution = 1/Fs;           % Step size of digital measurements
    
    % Biases
    
    %imu.Gyroscope.BiasInstability = 0.012 * 3.14159 / 180;       % rad/hr
    %imu.Gyroscope.NoiseDensity = 0.15 * 3.14159 / 180;          % rad/s
    %imu.Gyroscope.RandomWalk = 0.017 * 3.14159 / 180;           % rad/sqrt(hr)
    %imu.Gyroscope.TemperatureBias = 0.25 * 3.14159 / 180;       % rad/s
    %imu.Gyroscope.AccelerationBias = 0.3;
    
    % Define real accelerations
    %acc(:,1) = 1;
    [~, gyroData] = imu(acc, angvel, eye(3));
    
    wx = gyroData(1);
    wy = gyroData(2);
    wz = gyroData(3);

end

== matlab function AeroCoeffsNew/Subsystem1/MATLAB Function ==
  data: t input; u_0 output; u0 input; u1 input; u2 input; deltat input; u_1 output; u_2 output
function [u_0, u_1, u_2] = fcn(t, u0, u1, u2, deltat)

point = (t+deltat)/deltat;
point = round(point);
if point > length(u0)
    u_0 = u0(length(u0));
    u_1 = u1(length(u1));
    u_2 = u2(length(u2));
else
    u_0 = u0(point);
    u_1 = u1(point);
    u_2 = u2(point);
end

end

== matlab function AeroCoeffsNew/Subsystem5/MATLAB Function5 ==
  data: M_y input; F1 output; F_z input; F2 output; F3 output
function [F1, F2, F3] = fcn(M_y, F_z)
xt_1 = 1.2598;
xb_1 = 2.2598;
xt_3 = -1.3402;
x_t1 = xt_1;
x_b1 = xb_1;
x_t3 = xt_3;



A_mat = [1 1;
    xt_1 xb_1];

A_inv = inv(A_mat);

p_0 = 0.2;
p_minus1 = 0;
step = 1000;
Converged = 0;
p_list = [];
x_list = [];
y_list = [];
J_list = [];
Fzz =[];
Myy =[];
while Converged == 0
    B = [(F_z - 4*p_0); (M_y - 4*p_0*xt_3)];
    force_0 = (A_inv*B);
    J_0 = sqrt(force_0(1)^2 + force_0(2)^2 + p_0^2);
    back = A_mat*force_0;
    backtrack = [4*p_0; 4*p_0*xt_3];
    forceback = back+backtrack;
    diff = sum(abs(forceback - [F_z; M_y]));
    if diff > 10^(-7)
        disp('Error')
        break
    end
    force = force_0;
    J = J_0;
    p = p_0;
    
    p_1 = p_0 + step;
    B = [(F_z - 4*p_1); (M_y - 4*p_1*xt_3)];
    force_1 = (A_inv*B);
    J_1 = sqrt(force_1(1)^2 + force_1(2)^2 + p_1^2);
    back = A_mat*force_1;
    backtrack = [4*p_1; 4*p_1*xt_3];
    forceback = back+backtrack;
    diff = sum(abs(forceback - [F_z; M_y]));
    if diff > 10^(-7)
        disp('Error')
        break
    end
    if J_1 < J_0
        force = force_1;
        J = J_1;
        p = p_1;
    end
    
    p_2 = p_0 - step;
    B = [(F_z - 4*p_2); (M_y - 4*p_2*xt_3)];
    force_2 = (A_inv*B);
    J_2 = sqrt(force_2(1)^2 + force_2(2)^2 + p_2^2);
    back = A_mat*force_2;
    backtrack = [4*p_2; 4*p_2*xt_3];
    forceback = back+backtrack;
    diff = sum(abs(forceback - [F_z; M_y]));
    if diff > 10^(-7)
        disp('Error')
        break
    end
    if J_2 < J_0 && J_2 < J_1
        force = force_2;
        J = J_2;
        p = p_2;
    end
    
    if p_minus1 < p_0 && p_0 < p
        step = step;
    elseif p_minus1 > p_0 && p_0 > p
        step = step;
    else
        step = step*0.9;
    end
        
    p_minus1 = p_0;
    p_0 = p;
    p_list = [p_list; p_0];
    x_list = [x_list; force(1)];
    y_list = [y_list; force(2)];
    J_list = [J_list; J];
    if step < abs(min([F_z,M_y])*10^(-9))
        Converged = 1;
    end
    
    
end

F1 = x_list(length(x_list));
F2 = y_list(length(y_list));
F3 = p_0;
end
